simulink model "test_dynamics"  (R2017a)
settings: Solver=VariableStepAuto  StartTime=0.0  StopTime=1  MaxStep=1e-5  RelTol=1e-3
libraries: simulink x1, slidercrank_basic_library_v1 x1
settings Model: Creator=filip  LastModifiedBy=filip

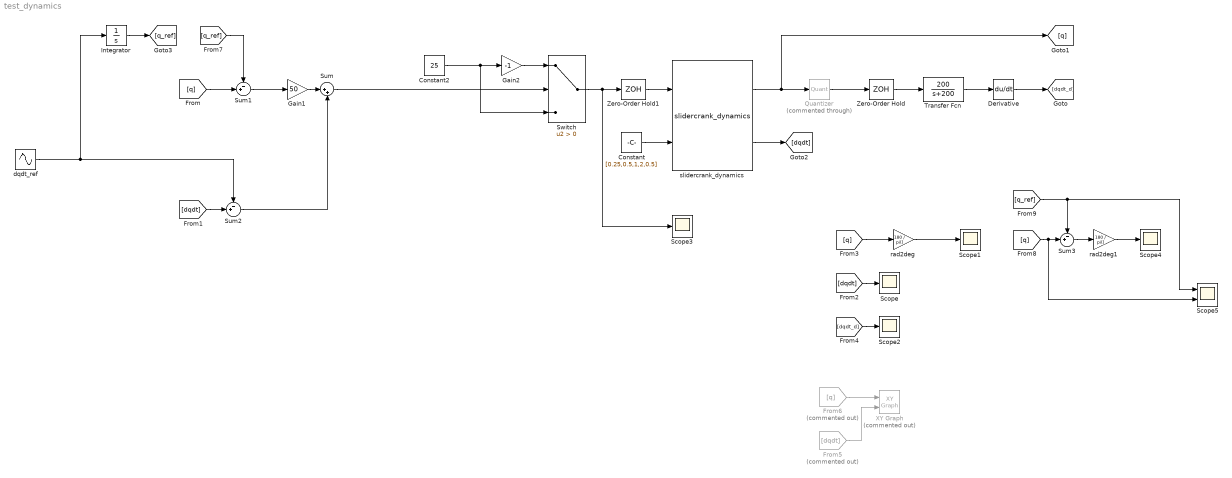
== system test_dynamics ==
  Constant : Constant  Value=[0.25,0.5,1,2,0.5]
  Constant2 : Constant  Value=25
  Derivative : Derivative  CoefficientInTFapproximation=1000
  From5 : From  Commented=on  GotoTag=dqdt
  From6 : From  Commented=on  GotoTag=q
  Gain1 : Gain  Gain=50
  Gain2 : Gain  Gain=-1
  Integrator : Integrator
  Quantizer : Quantizer  Commented=through  QuantizationInterval=2*pi()/4096
  Scope{,1..4} (5 alike) : Scope
  Scope5 : Scope  NumInputPorts=2
  Sum : Sum  Inputs=|++
  Sum1 : Sum  Inputs=-+|
  Sum2 : Sum  Inputs=-+|
  Sum3 : Sum  Inputs=-+|
  Switch : Switch  Criteria=u2 > Threshold
  Transfer Fcn : TransferFcn  Numerator=[200]  Denominator=[1 200]
  XY Graph : simulink/Sinks/XY Graph  Commented=on  xmin=-1  xmax=1  ymin=-60  ymax=60  st=1e-3
  Zero-Order Hold : ZeroOrderHold  SampleTime=1e-3
  Zero-Order Hold1 : ZeroOrderHold  SampleTime=1e-3
  dqdt_ref : Sin  Frequency=10  SampleTime=0
  rad2deg : Gain  Gain=180 / pi()
  rad2deg1 : Gain  Gain=180 / pi()
  slidercrank_dynamics : slidercrank_basic_library_v1/slidercrank_dynamics
  wires:
  Constant/1 -> slidercrank_dynamics/2
  slidercrank_dynamics/1 -> [q], Quantizer/1
  Quantizer/1 -> Zero-Order Hold/1
  Zero-Order Hold/1 -> Transfer Fcn/1
  Transfer Fcn/1 -> Derivative/1
  slidercrank_dynamics/2 -> [dqdt]
  Derivative/1 -> [dqdt_d]
  Constant2/1 -> Switch/3, Gain2/1
  Sum/1 -> Switch/2
  Zero-Order Hold1/1 -> slidercrank_dynamics/1
  Switch/1 -> Scope3/1, Zero-Order Hold1/1
  Gain2/1 -> Switch/1
  [dqdt] -> Scope/1
  [q] -> rad2deg/1
  [dqdt_d] -> Scope2/1
  rad2deg/1 -> Scope1/1
  From6/1 -> XY Graph/1
  From5/1 -> XY Graph/2
  Gain1/1 -> Sum/1
  Sum1/1 -> Gain1/1
  [q] -> Sum1/2
  [dqdt] -> Sum2/2
  dqdt_ref/1 -> Integrator/1, Sum2/1
  Sum2/1 -> Sum/2
  Integrator/1 -> [q_ref]
  [q_ref] -> Sum1/1
  [q] -> Scope5/2, Sum3/2
  Sum3/1 -> rad2deg1/1
  rad2deg1/1 -> Scope4/1
  [q_ref] -> Scope5/1, Sum3/1
